simulink model "ipmsm_velocity_control_system_coupler"  (R2022a)
settings: Solver=daessc  StartTime=0.0  StopTime=SimStopTime  FixedStep=Ts  RelTol=1e-3  AbsTol=1e-3
values from neighbouring files (symbols this model uses):
  battery_pack_TimeStep = 0.01    [PMSM_system_data.sldd]
  Ts = 5.0E-6    [PMSM_system_data.sldd]
  V_init = 377.0    [PMSM_plant_parameters.sldd]
undefined symbols (not defined in the file or in its folder): DiscIntNeverNeededParam, iabc, rotation_speed, Tq, V_dc
libraries: fl_lib x20, nesl_utility x20, ee_lib x4, simulink x1, eePwmGeneratorTwoLevel x1, SignalEditorBlockLib x1
Description:
  | IPMSM Velocity Control
settings Model: DataDictionary=PMSM_system_data.sldd  Creator=The MathWorks, Inc.  LastModifiedBy=tshintai
settings SolverCC: AutoScaleAbsTol=off  AlgebraicLoopSolver=TrustRegion
settings DataIOCC: MaxDataPoints=210000  DSMLogging=off  SignalLoggingName=logsout_ee_ipmsm_velocity_control
settings OptimizationCC: LifeSpan=inf
settings DebuggingCC: UnderspecifiedInitializationDetection=Classic  MergeDetectMultiDrivingBlocksExec=none  ParameterPrecisionLossMsg=none  UnconnectedInputMsg=warning  UnconnectedOutputMsg=warning  UnconnectedLineMsg=warning  SFUnexpectedBacktrackingDiag=warning  SFNoUnconditionalDefaultTransitionDiag=warning  SFExecutionAtInitializationDiag=none  SFMachineParentedDataDiag=warning  ArithmeticOperatorsInVariantConditions=warning
settings SFSimCC: SimUseLocalCustomCode=off  CustomCodeUndefinedFunction=UseInterfaceOnly
settings RTWCC: RTWUseLocalCustomCode=off  DLArmComputeVersion=19.05
settings CodeAppCC: StateflowObjectComments=on
settings GRTTargetCC: TargetLangStandard=C89/C90 (ANSI)
settings ConfigComp: CovMetricSettings=dw  CovSaveCumulativeToWorkspaceVar=on  CovSaveSingleToWorkspaceVar=on  CovExternalEMLEnable=off
settings SimscapeCC: SimscapeNormalizeSystem=off  SimscapeLogType=all  SimscapeLogToSDI=on  SimscapeLogName=simlog_ee_ipmsm_velocity_control  SimscapeLogLimitData=off  SimscapeLogDataHistory=210000

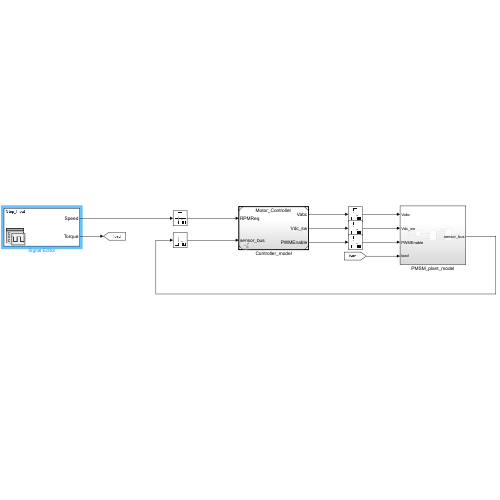
[thumbnail: Simulink's stored preview of the top-level diagram]
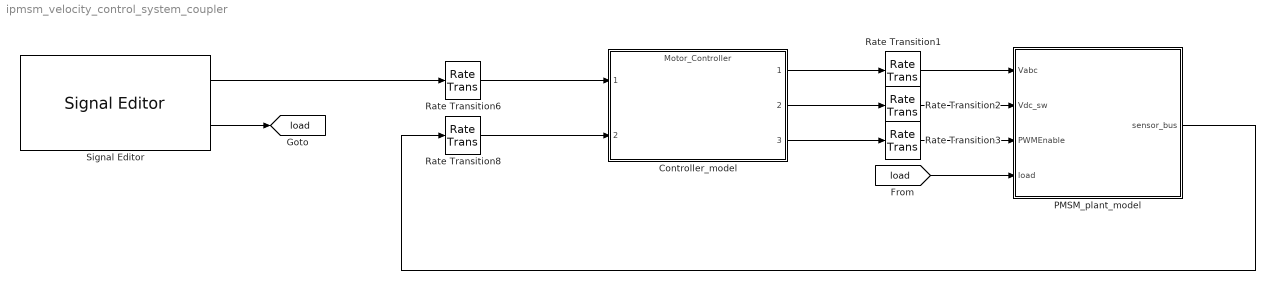
== system ipmsm_velocity_control_system_coupler ==
  Controller_model : ModelReference  ModelNameDialog=Motor_Controller.slx  SimulationMode=Normal  ModelReferenceVersion=4.3
  PMSM_plant_model : Subsystem
  Rate Transition1 : RateTransition
  Rate Transition2 : RateTransition
  Rate Transition3 : RateTransition
  Rate Transition6 : RateTransition  OutPortSampleTime=Tso
  Rate Transition8 : RateTransition  OutPortSampleTime=Tsi
  Signal Editor : SignalEditorBlockLib/Signal Editor  FileName=Motor_Controller_sig.mat  ActiveScenario=Step_Input  ActiveSignal=Speed  IsBus=off  OutputBusObjectStr=Bus: BusObject  SampleTime=0  ZeroCross=off  OutputAfterFinalValue=Holding final value  Unit=inherit  PreserveSignalName=on
  tag scope: load=global
  wires:
  Controller_model/1 -> Rate Transition1/1
  Signal Editor/2 -> [load]
  Signal Editor/1 -> Rate Transition6/1
  Rate Transition1/1 -> PMSM_plant_model/1(Vabc)
  Controller_model/2 -> Rate Transition2/1
  Rate Transition2/1 -> PMSM_plant_model/2(Vdc_sw)
  Rate Transition3/1 -> PMSM_plant_model/3(PWMEnable)
  Controller_model/3 -> Rate Transition3/1
  Rate Transition6/1 -> Controller_model/1
  [load] -> PMSM_plant_model/4(load)
  Rate Transition8/1 -> Controller_model/2
  PMSM_plant_model/1(sensor_bus) -> Rate Transition8/1

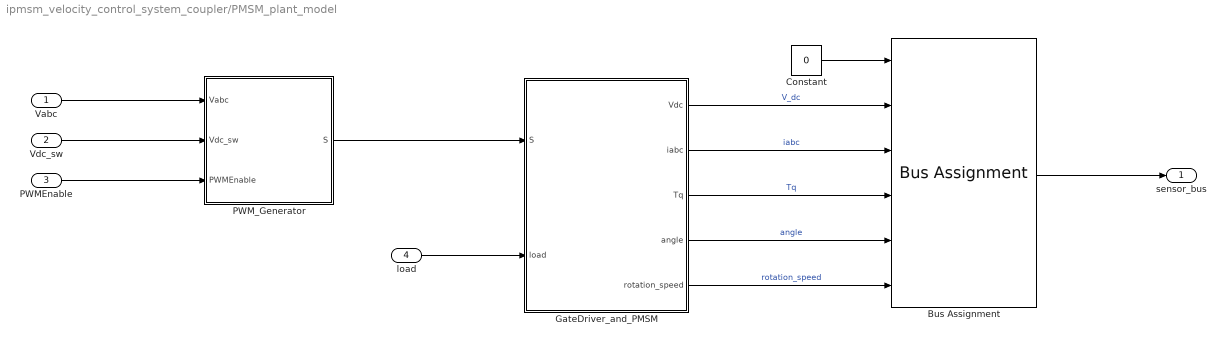
== system ipmsm_velocity_control_system_coupler/PMSM_plant_model ==
  Vabc : Inport
  Vdc_sw : Inport  Port=2
  PWMEnable : Inport  Port=3
  load : Inport  Port=4
  Bus Assignment : BusAssignment  AssignedSignals=V_dc,iabc,Tq,angle,rotation_speed
  Constant : Constant  Value=0  OutDataTypeStr=Bus: sensor_bus
  GateDriver_and_PMSM : Subsystem
  PWM_Generator : Subsystem
  sensor_bus : Outport
  wires:
  Vabc/1 -> PWM_Generator/1(Vabc)
  Vdc_sw/1 -> PWM_Generator/2(Vdc_sw)
  PWMEnable/1 -> PWM_Generator/3(PWMEnable)
  PWM_Generator/1(S) -> GateDriver_and_PMSM/1(S)
  load/1 -> GateDriver_and_PMSM/2(load)
  GateDriver_and_PMSM/1(Vdc) -> Bus Assignment/2  "V_dc"
  GateDriver_and_PMSM/2(iabc) -> Bus Assignment/3  "iabc"
  GateDriver_and_PMSM/3(Tq) -> Bus Assignment/4  "Tq"
  GateDriver_and_PMSM/4(angle) -> Bus Assignment/5  "angle"
  GateDriver_and_PMSM/5(rotation_speed) -> Bus Assignment/6  "rotation_speed"
  Constant/1 -> Bus Assignment/1
  Bus Assignment/1 -> sensor_bus/1

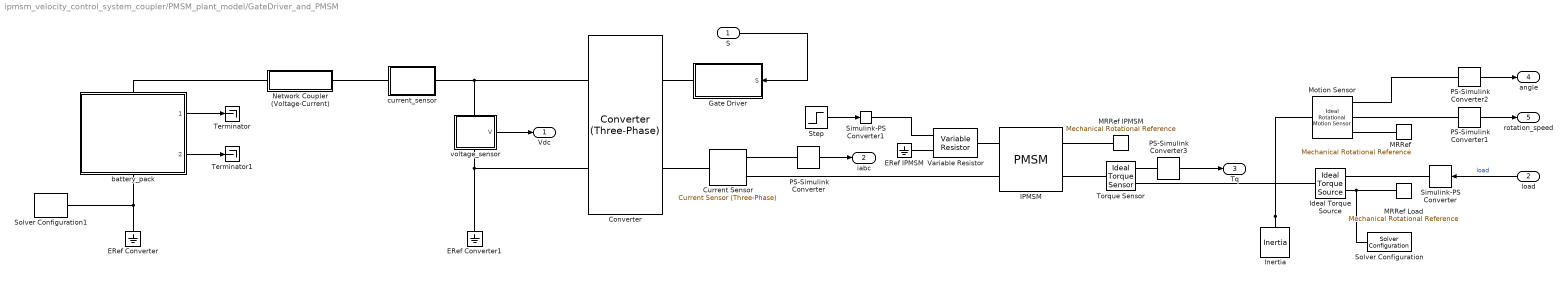
== system ipmsm_velocity_control_system_coupler/PMSM_plant_model/GateDriver_and_PMSM ==
  S : Inport
  load : Inport  Port=2
  Converter : ee_lib/Semiconductors & Converters/Converters/Converter (Three-Phase)  port_option=ee.enum.threePhasePort.composite  device_type=3  Vf=0.8 V  Ron=0.001 Ohm  Rds=0.001 Ohm  Goff=1e-5 1/Ohm  Vgt=1 V  Vgt_off=-1 V  Ih=1 A  Vth=0.5 V  diode_param=2  diode_Vf=0.8 V  diode_Ron=0.001 Ohm  diode_Goff=1e-5 1/Ohm  diode_C=50 nF  diode_iRM=-235 A  diode_iF=300 A  diode_idot=-50 A/us  diode_trr_param=1  diode_trr_factor=3  diode_trr=15 us  diode_Qrr=1.5e+3 s*uA  snubber_type=0  Cs=1e-7 F  Rs=0.1 Ohm
      settings: SourceProductBaseCode=PS
  Current Sensor : ee_lib/Sensors & Transducers/Current Sensor (Three-Phase)
  ERef Converter : fl_lib/Electrical/Electrical Elements/Electrical Reference
      settings: SourceProductBaseCode=PW,SS,VE
  ERef Converter1 : fl_lib/Electrical/Electrical Elements/Electrical Reference
      settings: SourceProductBaseCode=PW,SS,VE
  ERef IPMSM : fl_lib/Electrical/Electrical Elements/Electrical Reference
      settings: SourceProductBaseCode=PW,SS,VE
  Gate Driver : Subsystem
  IPMSM : ee_lib/Electromechanical/Permanent Magnet/PMSM  port_option=ee.enum.threePhasePort.composite  winding_type=ee.enum.statorconnection.wye  machine_param=ee.enum.pmsm.parameterization.constant  nPolePairs=p  pmflux_param=1  pm_flux_linkage=psim Wb  torque_constant=0.18 N*m/A  back_emf_constant=0.18 V/(rad/s)  stator_param=1  Ld=Ld H  Lq=Lq H  idVec=[-200, 0, 200] A  iqVec=[-200, 0, 200] A  LdMatrix=0.0002 * ones(3, 3) H  LqMatrix=0.0002 * ones(3, 3) H  PmMatrix=0.1 * ones(3, 3) Wb  ktMatrix=0.18 * ones(3, 3) N*m/A  keMatrix=0.18 * ones(3, 3) V/(rad/s)  L0=L0 H  Ls=0.0002 H  Lm=0.00002 H  Ms=0.00002 H  Rs=Rs Ohm  zero_sequence=ee.enum.park.zerosequence.include  axes_param=1  loss_param=ee.enum.ironloss.none  losses_oc=[0, 0, 0] W  losses_sc=[0, 0, 0] W  f_losses=60 Hz  Isc_losses=95 A  J=0 kg*m^2  lam=0 N*m/(rad/s)  i_d_specify=off  i_d_priority=None  i_d=0 A  i_d_nominal_specify=off  i_d_nominal_unit=A  i_d_nominal_value=1  i_q_specify=off  i_q_priority=None  i_q=0 A  i_q_nominal_specify=off  i_q_nominal_unit=A  i_q_nominal_value=1  torque_specify=off  torque_priority=None  torque=0 N*m  torque_nominal_specify=off  torque_nominal_unit=N*m  torque_nominal_value=1  angular_velocity_specify=on  angular_velocity_priority=None  angular_velocity=0 rpm  angular_velocity_nominal_specify=off  angular_velocity_nominal_unit=rpm  angular_velocity_nominal_value=1  angular_position_specify=on  angular_position_priority=High  angular_position=0 rad  angular_position_nominal_specify=off  angular_position_nominal_unit=deg  angular_position_nominal_value=1  alpha=3.93e-3 1/K  alpha_flux=-0.001 1/K  Tmeas=298.15 K  stator_thermal_mass=100 J/K  rotor_thermal_mass=200 J/K  Rm_percent_rotor=90  Rd_percent_rotor=30  temperatureA_specify=off  temperatureA_priority=High  temperatureA=25 degC  temperatureA_nominal_specify=off  temperatureA_nominal_unit=degC  temperatureA_nominal_value=1  temperatureB_specify=off  temperatureB_priority=High  temperatureB=25 degC  temperatureB_nominal_specify=off  temperatureB_nominal_unit=degC  temperatureB_nominal_value=1  temperatureC_specify=off  temperatureC_priority=High  temperatureC=25 degC  temperatureC_nominal_specify=off  temperatureC_nominal_unit=degC  temperatureC_nominal_value=1  temperatureR_specify=off  temperatureR_priority=High  temperatureR=25 degC  temperatureR_nominal_specify=off  temperatureR_nominal_unit=degC  temperatureR_nominal_value=1
      settings: AttributesFormatString=35 kW  InternalSimscapePortConfiguration="{\"Bottom\":[],\"Left\":[{\"id\":\"N\",\"label\":\"~\",\"type\":\"foundation.electrical.three_phase\"},{\"id\":\"n\",\"label\":\"n\",\"type\":\"foundation.electrical.electrical\"}],\"Right\":[{\"id\":\"R\",\"label\":\"R\",\"type\":\"foundation.mechanical.rotational.rotational\"},{\"id\":\"C\",\"label\":\"C\",\"type\":\"foundation.mechanical.rotational.rotational\"}],\"Top\":[]}"
  Ideal Torque Source : fl_lib/Mechanical/Mechanical Sources/Ideal Torque Source
      settings: SourceProductBaseCode=PW,SS,VE
  Inertia : fl_lib/Mechanical/Rotational Elements/Inertia  inertia=Jm kg*m^2  num_ports=foundation.enum.numPorts2.one  w_specify=on  w_priority=High  w=0 rpm  w_nominal_specify=off  w_nominal_unit=rad/s  w_nominal_value=1  t_specify=off  t_priority=High  t=0 N*m  t_nominal_specify=off  t_nominal_unit=N*m  t_nominal_value=1
      settings: SourceProductBaseCode=PW,SS,VE
  MRRef : fl_lib/Mechanical/Rotational Elements/Mechanical Rotational Reference
      settings: SourceProductBaseCode=PW,SS,VE
  MRRef IPMSM : fl_lib/Mechanical/Rotational Elements/Mechanical Rotational Reference
      settings: SourceProductBaseCode=PW,SS,VE
  MRRef Load : fl_lib/Mechanical/Rotational Elements/Mechanical Rotational Reference
      settings: SourceProductBaseCode=PW,SS,VE
  Motion Sensor : fl_lib/Mechanical/Mechanical Sensors/Ideal Rotational Motion Sensor  wrap_angle=simscape.enum.onoff.off  offset=0 deg
      settings: SourceProductBaseCode=PW,SS,VE
  Network Coupler (Voltage-Current) : Subsystem  mask(Network Coupler (Voltage-Current)){}
      mask init:
      | % Icon
      | key = 'Simscape.NetworkCouplers.ElectricalVoltageCurrent';
      | foundation.internal.couplers.updateIcon(gcb,'voltageCurrentSource.svg',key)
      settings: OpenFcn=open_system(gcbh,'force')
      mask Help: web([docroot '/physmod/simscape/ref/networkcouplervoltagecurrent.html'])
      mask Display:
      | color('red');
      | port_label('LConn', 1,'1')
      | port_label('RConn', 1,'2')
  PS-Simulink Converter : nesl_utility/PS-Simulink Converter  PhysicalDomain=network_engine_domain  SubClassName=ps_output  LeftPortType=input  RightPortType=output  PseudoPeriodic=off  Frequencies=[]  VectorFormat=1-D array  Unit=A  AffineConversion=off
      settings: SourceProductBaseCode=SS,PW,VE
  PS-Simulink Converter1 : nesl_utility/PS-Simulink Converter  PhysicalDomain=network_engine_domain  SubClassName=ps_output  LeftPortType=input  RightPortType=output  PseudoPeriodic=off  Frequencies=[]  VectorFormat=1-D array  Unit=rad/s  AffineConversion=off
      settings: SourceProductBaseCode=SS,PW,VE
  PS-Simulink Converter2 : nesl_utility/PS-Simulink Converter  PhysicalDomain=network_engine_domain  SubClassName=ps_output  LeftPortType=input  RightPortType=output  PseudoPeriodic=off  Frequencies=[]  VectorFormat=1-D array  Unit=rad  AffineConversion=off
      settings: SourceProductBaseCode=SS,PW,VE
  PS-Simulink Converter3 : nesl_utility/PS-Simulink Converter  PhysicalDomain=network_engine_domain  SubClassName=ps_output  LeftPortType=input  RightPortType=output  PseudoPeriodic=off  Frequencies=[]  VectorFormat=1-D array  Unit=N*m  AffineConversion=off
      settings: SourceProductBaseCode=SS,PW,VE
  Simulink-PS Converter : nesl_utility/Simulink-PS Converter  PhysicalDomain=network_engine_domain  SubClassName=ps_input  LeftPortType=input  RightPortType=output  PseudoPeriodic=off  Frequencies=[]  NoiseDistribution=none  NoiseParameters=[]  Unit=N*m  AffineConversion=off  FilteringAndDerivatives=zero  SimscapeFilterOrder=1  InputFilterTimeConstant=0.001  UdotUserProvided=1
      settings: SourceProductBaseCode=SS,PW,VE
  Simulink-PS Converter1 : nesl_utility/Simulink-PS Converter  PhysicalDomain=network_engine_domain  SubClassName=ps_input  LeftPortType=input  RightPortType=output  PseudoPeriodic=off  Frequencies=[]  NoiseDistribution=none  NoiseParameters=[]  Unit=1  AffineConversion=off  FilteringAndDerivatives=provide  SimscapeFilterOrder=1  InputFilterTimeConstant=0.001  UdotUserProvided=0
      settings: SourceProductBaseCode=SS,PW,VE
  Solver Configuration : nesl_utility/Solver Configuration  PhysicalDomain=network_engine_domain  SubClassName=solver  LeftPortType=input  RightPortType=generic  Tones=[]  Harmonics=[]  SimulateNoise=off  Profile=off  UseLocalSampling=off  EnableSwitchedLinearOptims=on  FrequencyDomain=off  UseCCode=off  RelTol=0.001  AbsTol=1e-06  MinStep=1e-09  ToWorkspace=off  RevertToSquareIcSolve=off  NumHomotopyIterations=100  PhasorMode=off  PhasorModeNumHarmonics=1  IndexReductionMethod=DerivativeReplacement  DoDC=off  ResidualTolerance=1e-9  UseLocalSolver=on  LocalSolverChoice=NE_BACKWARD_EULER_ADVANCER  LocalSolverSampleTime=Ts  DoFixedCost=on  MaxNonlinIter=5  MaxModeIter=2  ComputeImpulses=off  ImpulseIterations=2  LinearAlgebra=auto  LinearAlgebraNumThread=0  EquationFormulation=NE_TIME_EF  DelaysMemoryBudget=1024  AutomaticFiltering=on  FilteringTimeConstant=0.001  PartitionStorageMethod=AS_NEEDED  PartitionMemoryBudget=1024  PartitionMethod=FAST
      settings: SourceProductBaseCode=SS,PW,VE
  Solver Configuration1 : nesl_utility/Solver Configuration  PhysicalDomain=network_engine_domain  SubClassName=solver  LeftPortType=input  RightPortType=generic  Tones=[]  Harmonics=[]  SimulateNoise=off  Profile=off  UseLocalSampling=off  EnableSwitchedLinearOptims=on  FrequencyDomain=off  UseCCode=off  RelTol=0.001  AbsTol=0.001  MinStep=1e-09  ToWorkspace=off  RevertToSquareIcSolve=off  NumHomotopyIterations=100  PhasorMode=off  PhasorModeNumHarmonics=1  IndexReductionMethod=DerivativeReplacement  DoDC=off  ResidualTolerance=1e-09  UseLocalSolver=on  LocalSolverChoice=NE_BACKWARD_EULER_ADVANCER  LocalSolverSampleTime=battery_pack_TimeStep  DoFixedCost=on  MaxNonlinIter=3  MaxModeIter=2  ComputeImpulses=off  ImpulseIterations=2  LinearAlgebra=auto  LinearAlgebraNumThread=0  EquationFormulation=NE_TIME_EF  DelaysMemoryBudget=1024  AutomaticFiltering=on  FilteringTimeConstant=0.001  PartitionStorageMethod=AS_NEEDED  PartitionMemoryBudget=1024  PartitionMethod=ROBUST
      settings: SourceProductBaseCode=SS,PW,VE
  Step : Step  Time=0.3  Before=1e9  After=1e9  SampleTime=0
  Terminator : Terminator
  Terminator1 : Terminator
  Torque Sensor : fl_lib/Mechanical/Mechanical Sensors/Ideal Torque Sensor
      settings: SourceProductBaseCode=PW,SS,VE
  Variable Resistor : fl_lib/Electrical/Electrical Elements/Variable Resistor  Rmin=0 Ohm  i_specify=off  i_priority=None  i=0 A  i_nominal_specify=off  i_nominal_unit=A  i_nominal_value=1  v_specify=off  v_priority=None  v=0 V  v_nominal_specify=off  v_nominal_unit=V  v_nominal_value=1
      settings: SourceProductBaseCode=PW,SS,VE
  battery_pack : Subsystem  ReferencedSubsystem=battery_96_pack
      settings: PortSchema="{\"entries\":[{\"content\":{\"sides\":[{\"content\":{\"connectorIds\":[]},\"type\":\"ConnectorPlacement.EquallySpacedRectSide\",\"uuid\":\"485b780b-fec5-4a6e-9c4a-84b4d939a40e\"},{\"content\":{\"connectorIds\":[\"Out1\",\"Out2\"],\"side\":\"RIGHT\"},\"type\":\"ConnectorPlacement.EquallySpacedRectSide\",\"uuid\":\"e63a9d0c-46b2-44d5-a80a-3c6cfd714558\"},{\"content\":{\"connectorIds\":[\"LConn1\"],\"side\":\"TOP\"},\"type\":\"ConnectorPlacement.EquallySpacedRectSide\",\"uuid\":\"fa88f5e9-c256-49a0-983f-41440d45b27d\"},{\"content\":{\"connectorIds\":[\"RConn1\"],\"side\":\"BOTTOM\"},\"type\":\"ConnectorPlacement.EquallySpacedRectSide\",\"uuid\":\"af720e83-a3fc-4197-ae0f-d9d0aa453c8d\"}]},\"type\":\"ConnectorPlacement.EquallySpacedConnector\",\"uuid\":\"f46161be-ef35-45f2-922c-6cbb80c1717a\"}],\"packageUris\":[\"http://schema.mathworks.com/mf0/Connector/R2020b\"],\"version\":\"1.0\"}"
  current_sensor : Subsystem
  voltage_sensor : Subsystem
      settings: PortSchema="{\"entries\":[{\"content\":{\"sides\":[{\"content\":{\"connectorIds\":[]},\"type\":\"ConnectorPlacement.EquallySpacedRectSide\",\"uuid\":\"3cec5e81-2f0a-4a37-ad46-63204ea5d66a\"},{\"content\":{\"connectorIds\":[\"Out1\"],\"side\":\"RIGHT\"},\"type\":\"ConnectorPlacement.EquallySpacedRectSide\",\"uuid\":\"919246d8-ddc0-4701-8a0b-6f7af372975e\"},{\"content\":{\"connectorIds\":[\"LConn1\"],\"side\":\"TOP\"},\"type\":\"ConnectorPlacement.EquallySpacedRectSide\",\"uuid\":\"caca8a5a-fb83-489d-995f-a589d1d02c9f\"},{\"content\":{\"connectorIds\":[\"RConn1\"],\"side\":\"BOTTOM\"},\"type\":\"ConnectorPlacement.EquallySpacedRectSide\",\"uuid\":\"97d0da43-b632-476f-bdfd-058552dcf5f1\"}]},\"type\":\"ConnectorPlacement.EquallySpacedConnector\",\"uuid\":\"08c9aed4-62a1-4b8a-bec9-e16a3b517ce3\"}],\"packageUris\":[\"http://schema.mathworks.com/mf0/Connector/R2020b\"],\"version\":\"1.0\"}"
  Vdc : Outport
  iabc : Outport  Port=2
  Tq : Outport  Port=3
  angle : Outport  Port=4
  rotation_speed : Outport  Port=5
  wires:
  load/1 -> Simulink-PS Converter/1  "load"
  S/1 -> Gate Driver/1(S)
  PS-Simulink Converter/1 -> iabc/1
  PS-Simulink Converter2/1 -> angle/1
  PS-Simulink Converter1/1 -> rotation_speed/1
  PS-Simulink Converter3/1 -> Tq/1
  Step/1 -> Simulink-PS Converter1/1
  voltage_sensor/1(V) -> Vdc/1
  battery_pack/1 -> Terminator/1
  battery_pack/2 -> Terminator1/1
  connections:
  Variable Resistor/LConn2 -- ERef IPMSM/LConn1
  Ideal Torque Source/RConn1 -- Simulink-PS Converter/RConn1
  Variable Resistor/RConn1 -- IPMSM/LConn2
  Solver Configuration/RConn1 -- Ideal Torque Source/RConn2 -- MRRef Load/LConn1
  Gate Driver/RConn1 -- Converter/LConn1
  Torque Sensor/LConn1 -- IPMSM/RConn1
  Inertia/LConn1 -- Ideal Torque Source/LConn1 -- Torque Sensor/RConn1 -- Motion Sensor/LConn1
  Network Coupler (Voltage-Current)/LConn1 -- current_sensor/LConn1
  IPMSM/RConn2 -- MRRef IPMSM/LConn1
  Current Sensor/RConn1 -- PS-Simulink Converter/LConn1
  IPMSM/LConn1 -- Current Sensor/RConn2
  Converter/LConn2 -- Current Sensor/LConn1
  Motion Sensor/RConn2 -- PS-Simulink Converter1/LConn1
  Motion Sensor/RConn3 -- PS-Simulink Converter2/LConn1
  MRRef/LConn1 -- Motion Sensor/RConn1
  Torque Sensor/RConn2 -- PS-Simulink Converter3/LConn1
  Converter/RConn2 -- ERef Converter1/LConn1 -- voltage_sensor/RConn1
  Simulink-PS Converter1/RConn1 -- Variable Resistor/LConn1
  Converter/RConn1 -- voltage_sensor/LConn1 -- current_sensor/RConn1
  Network Coupler (Voltage-Current)/RConn1 -- battery_pack/LConn1
  Solver Configuration1/RConn1 -- ERef Converter/LConn1 -- battery_pack/RConn1

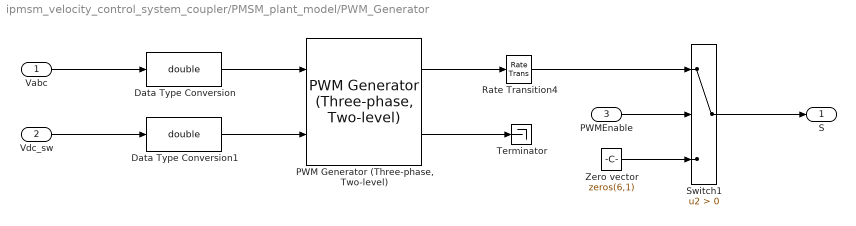
== system ipmsm_velocity_control_system_coupler/PMSM_plant_model/PWM_Generator ==
  Vabc : Inport
  Vdc_sw : Inport  Port=2
  PWMEnable : Inport  Port=3
  Data Type Conversion : DataTypeConversion  OutDataTypeStr=double  SaturateOnIntegerOverflow=off  RndMeth=Floor
  Data Type Conversion1 : DataTypeConversion  OutDataTypeStr=double  SaturateOnIntegerOverflow=off  RndMeth=Floor
  "PWM Generator (Three-phase, Two-level)" : eePwmGeneratorTwoLevel/PWM Generator (Three-phase, Two-level)  PWMMode=Continuous PWM (CPWM)  CPWMMode=SVM: space vector modulation  DPWMMode=60 DPWM: 60 degree discontinuous PWM  fsw=fsw  Ts=Ts
      settings: SourceProductBaseCode=PS
  Rate Transition4 : RateTransition
  Switch1 : Switch  Criteria=u2 > Threshold  SaturateOnIntegerOverflow=off  InputSameDT=off
  Terminator : Terminator
  Zero vector : Constant  Value=zeros(6,1)
  S : Outport
  wires:
  "PWM Generator (Three-phase, Two-level)"/2 -> Terminator/1
  Vabc/1 -> Data Type Conversion/1
  Zero vector/1 -> Switch1/3
  PWMEnable/1 -> Switch1/2
  Vdc_sw/1 -> Data Type Conversion1/1
  Rate Transition4/1 -> Switch1/1
  "PWM Generator (Three-phase, Two-level)"/1 -> Rate Transition4/1
  Switch1/1 -> S/1
  Data Type Conversion/1 -> "PWM Generator (Three-phase, Two-level)"/1
  Data Type Conversion1/1 -> "PWM Generator (Three-phase, Two-level)"/2

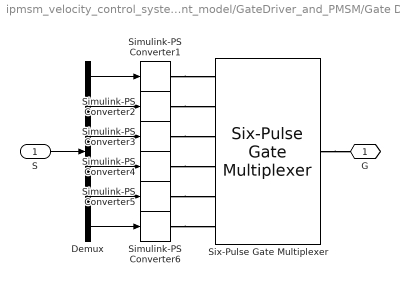
== system ipmsm_velocity_control_system_coupler/PMSM_plant_model/GateDriver_and_PMSM/Gate Driver ==
  S : Inport
  Demux : Demux  Outputs=6
  Simulink-PS Converter{1..6} (6 alike) : nesl_utility/Simulink-PS Converter  PhysicalDomain=network_engine_domain  SubClassName=ps_input  LeftPortType=input  RightPortType=output  PseudoPeriodic=off  Frequencies=[]  NoiseDistribution=none  NoiseParameters=[]  Unit=1  AffineConversion=off  FilteringAndDerivatives=zero  SimscapeFilterOrder=1  InputFilterTimeConstant=0.001  UdotUserProvided=1
      settings: SourceProductBaseCode=SS,PW,VE
  Six-Pulse Gate Multiplexer : ee_lib/Semiconductors & Converters/Converters/Six-Pulse Gate Multiplexer  port_option=ee.enum.controlport.ps
      settings: SourceProductBaseCode=PS
  G : PMIOPort  Side=Right
  wires:
  Demux/1 -> Simulink-PS Converter1/1
  S/1 -> Demux/1
  Demux/4 -> Simulink-PS Converter4/1
  Demux/2 -> Simulink-PS Converter2/1
  Demux/3 -> Simulink-PS Converter3/1
  Demux/5 -> Simulink-PS Converter5/1
  Demux/6 -> Simulink-PS Converter6/1
  connections:
  Six-Pulse Gate Multiplexer/RConn1 -- G/RConn1
  Simulink-PS Converter1/RConn1 -- Six-Pulse Gate Multiplexer/LConn1
  Simulink-PS Converter3/RConn1 -- Six-Pulse Gate Multiplexer/LConn3
  Simulink-PS Converter5/RConn1 -- Six-Pulse Gate Multiplexer/LConn5
  Simulink-PS Converter6/RConn1 -- Six-Pulse Gate Multiplexer/LConn6
  Simulink-PS Converter4/RConn1 -- Six-Pulse Gate Multiplexer/LConn4
  Simulink-PS Converter2/RConn1 -- Six-Pulse Gate Multiplexer/LConn2

== system ipmsm_velocity_control_system_coupler/PMSM_plant_model/GateDriver_and_PMSM/Network Coupler (Voltage-Current) ==
  note: Connect Port 1 to the network
      | with the smaller sample time, or
      | the network running variable step.
  note: Uncomment rate transition
      | blocks if one or both networks
      | are running fixed step.
  Port 1 Interface : Subsystem  mask(Network Coupler (Voltage-Current) Port 1 Interface){samplingType=Fixed step both ports with faster sampling at port 1, ts=1e-3, h1=Ts, h2=battery_pack_TimeStep, predictionDiscreteToContinuous=off, smoothingContinuousToDiscrete=off, predictionSlowToFast=off, smoothingFastToSlow=off, nSmooth=1, tsSmoothing=0.01, tsMax=0.5, tau=0.1, i0=0, v0=V_init}
      mask prompts: samplingType "physmod:simscape:couplers:SimscapeNetworkCouplersLib:SamplingType_MP"; ts "physmod:simscape:couplers:SimscapeNetworkCouplersLib:SeparatorTimeConstants_MP"; h1 "physmod:simscape:couplers:SimscapeNetworkCouplersLib:Port1NetworkDiscreteSampleTimes_MP"; h2 "physmod:simscape:couplers:SimscapeNetworkCouplersLib:Port2NetworkDiscreteSampleTimes_MP"; predictionDiscreteToContinuous "physmod:simscape:couplers:SimscapeNetworkCouplersLib:UsePredictionWhenConnectingFixedStepToVariableStep_MP"; smoothingContinuousToDiscrete "physmod:simscape:couplers:SimscapeNetworkCouplersLib:UseSmoothingWhenConnectingVariableStepToFixedStep_MP"; predictionSlowToFast "physmod:simscape:couplers:SimscapeNetworkCouplersLib:UsePredictionWhenConnectingSlowToFastSampleTimes_MP"; smoothingFastToSlow "physmod:simscape:couplers:SimscapeNetworkCouplersLib:UseSmoothingWhenConnectingFastToSlowSampleTimes_MP"; nSmooth "physmod:simscape:couplers:SimscapeNetworkCouplersLib:NumberOfSamplesOverWhichToSmooth_MP"; tsSmoothing "physmod:simscape:couplers:SimscapeNetworkCouplersLib:SmoothingTimeConstants_MP"; tsMax "physmod:simscape:couplers:SimscapeNetworkCouplersLib:CalculatedFastestTrackableTimeConstants_MP"; tau "physmod:simscape:couplers:SimscapeNetworkCouplersLib:CalculatedFilterTimeConstants_MP"; i0 "physmod:simscape:couplers:SimscapeNetworkCouplersLib:InitialCurrentA_MP"; v0 "physmod:simscape:couplers:SimscapeNetworkCouplersLib:InitialVoltageV_MP"
      mask help:
      | Port 1 interface for use when breaking two Simscape(TM) networks at an electrical connection. A first-order filter is used to break algebraic constraints between the two networks.
      |
      | Connect Port 1 to the network with the higher sample rate, or the network that is variable step if interfacing fixed step and variable step networks.
      mask init:
      | % Fixed step sample time value check
      | foundation.internal.couplers.checkSampleTimes(gcb,h1,h2);
      | 
      | % Derived parameters
      | [tau,tsMax] = foundation.internal.couplers.electrical.derivedParamsSources(gcb,ts,h1,h2);
      settings: PortSchema="{\"entries\":[{\"content\":{\"sides\":[{\"content\":{\"connectorIds\":[\"LConn1\"]},\"type\":\"ConnectorPlacement.EquallySpacedRectSide\",\"uuid\":\"a6d4a9fd-b5aa-40dc-ab7e-2b646b9b57bc\"},{\"content\":{\"connectorIds\":[\"Out1\",\"In1\"],\"side\":\"RIGHT\"},\"type\":\"ConnectorPlacement.EquallySpacedRectSide\",\"uuid\":\"31bb6273-5b9b-48d0-a1a2-6fbacb979b97\"},{\"content\":{\"connectorIds\":[],\"side\":\"TOP\"},\"type\":\"ConnectorPlacement.EquallySpacedRectSide\",\"uuid\":\"0f7afab2-4481-486c-9ad0-2b42c5b091a4\"}]},\"type\":\"ConnectorPlacement.EquallySpacedConnector\",\"uuid\":\"a98e47aa-cbfd-441a-b14c-c9ea515c056e\"}],\"packageUris\":[\"http://schema.mathworks.com/mf0/Connector/R2020b\"],\"version\":\"1.0\"}"
      mask Help: web([docroot '/physmod/simscape/ref/networkcouplervoltagecurrent.html'])
      mask TypeOptions samplingType: physmod:simscape:couplers:SimscapeNetworkCouplersLib:VariableStepAtPorts1And2_PV | physmod:simscape:couplers:SimscapeNetworkCouplersLib:VariableStepAtPort1AndFixedStepAtPort2_PV | physmod:simscape:couplers:SimscapeNetworkCouplersLib:FixedStepBothPortsWithCommonSampleTime_PV | physmod:simscape:couplers:SimscapeNetworkCouplersLib:FixedStepBothPortsWithFasterSamplingAtPort1_PV
      mask Callback samplingType: foundation.internal.couplers.electrical.parameterVisibilitiesSources(gcb)
      mask Callback predictionDiscreteToContinuous: foundation.internal.couplers.electrical.parameterVisibilitiesSources(gcb)
      mask Callback smoothingContinuousToDiscrete: foundation.internal.couplers.electrical.parameterVisibilitiesSources(gcb)
      mask Callback predictionSlowToFast: foundation.internal.couplers.electrical.parameterVisibilitiesSources(gcb)
      mask Callback smoothingFastToSlow: foundation.internal.couplers.electrical.parameterVisibilitiesSources(gcb)
      mask DialogControl Main Prompt: Main
      mask DialogControl samplingType Prompt: サンプリング タイプ
      mask DialogControl ts Prompt: 区切り時定数 (s)
      mask DialogControl h1 Prompt: 端子 1 のネットワークの離散サンプル時間 (s)
      mask DialogControl h2 Prompt: 端子 2 のネットワークの離散サンプル時間 (s)
      mask DialogControl predictionDiscreteToContinuous Prompt: 固定ステップを可変ステップに接続するときに予測を使用
      mask DialogControl smoothingContinuousToDiscrete Prompt: 可変ステップを固定ステップに接続するときに平滑化を使用
      mask DialogControl predictionSlowToFast Prompt: 低速のサンプル時間を高速のサンプル時間に接続するときに予測を使用
      mask DialogControl smoothingFastToSlow Prompt: 高速のサンプル時間を低速のサンプル時間に接続するときに平滑化を使用
      mask DialogControl nSmooth Prompt: 平滑化するサンプルの数
      mask DialogControl tsSmoothing Prompt: 平滑化時定数 (s)
      mask DialogControl Analysis Prompt: Analysis
      mask DialogControl tsMax Prompt: 計算された最速の追跡可能な時定数 (s)
      mask DialogControl tau Prompt: 計算されたフィルター時定数 (s)
      mask DialogControl updateRecommendations Prompt: Update
      mask DialogControl updateRecommendations Callback: foundation.internal.couplers.electrical.analysisSources(gcb);
      mask DialogControl InitialConditions Prompt: Initial Conditions
      mask DialogControl i0 Prompt: 初期電流 (A)
      mask DialogControl v0 Prompt: 初期電圧 (V)
  Port 2 Interface : Subsystem  mask(Network Coupler (Voltage-Current) Port 2 Interface){}
      mask help: physmod:simscape:couplers:SimscapeNetworkCouplersLib:NetworkCouplerVoltageCurrentPort2Interface_MD
      settings: PortSchema="{\"entries\":[{\"content\":{\"sides\":[{\"content\":{\"connectorIds\":[\"In1\",\"Out1\"]},\"type\":\"ConnectorPlacement.EquallySpacedRectSide\",\"uuid\":\"5a4c1550-e77d-42df-bf3e-b81963920de7\"},{\"content\":{\"connectorIds\":[\"RConn1\"],\"side\":\"RIGHT\"},\"type\":\"ConnectorPlacement.EquallySpacedRectSide\",\"uuid\":\"3fd730f7-5937-4563-a365-595aaae9027b\"},{\"content\":{\"connectorIds\":[],\"side\":\"TOP\"},\"type\":\"ConnectorPlacement.EquallySpacedRectSide\",\"uuid\":\"c16e04e4-26e8-4fd6-98d3-59adbef44c0d\"}]},\"type\":\"ConnectorPlacement.EquallySpacedConnector\",\"uuid\":\"5588d8d0-d459-45fe-a303-1ca6654e99d0\"}],\"packageUris\":[\"http://schema.mathworks.com/mf0/Connector/R2020b\"],\"version\":\"1.0\"}"
      mask Help: web([docroot '/physmod/simscape/ref/networkcouplervoltagecurrent.html'])
  Rate transition (fast-to-slow) : RateTransition  Commented=through  Integrity=off
  Rate transition (slow-to-fast) : RateTransition  Commented=through  Integrity=off
  1 : PMIOPort  Side=Left
  2 : PMIOPort  Port=2  Side=Right
  wires:
  Port 1 Interface/1(current) -> Rate transition (fast-to-slow)/1
  Rate transition (fast-to-slow)/1 -> Port 2 Interface/1(current)
  Port 2 Interface/1(voltage) -> Rate transition (slow-to-fast)/1
  Rate transition (slow-to-fast)/1 -> Port 1 Interface/1(voltage)
  connections:
  2/RConn1 -- Port 2 Interface/RConn1
  1/RConn1 -- Port 1 Interface/LConn1

== system ipmsm_velocity_control_system_coupler/PMSM_plant_model/GateDriver_and_PMSM/current_sensor ==
  Current Sensor1 : fl_lib/Electrical/Electrical Sensors/Current Sensor
      settings: SourceProductBaseCode=PW,SS,VE
  PS-Simulink Converter : nesl_utility/PS-Simulink Converter  PhysicalDomain=network_engine_domain  SubClassName=ps_output  LeftPortType=input  RightPortType=output  PseudoPeriodic=off  Frequencies=[]  VectorFormat=inherit  Unit=inherit  AffineConversion=off
      settings: SourceProductBaseCode=SS,PW,VE
  Terminator : Terminator
  + : PMIOPort  Side=Left
  - : PMIOPort  Port=2  Side=Right
  wires:
  PS-Simulink Converter/1 -> Terminator/1  "Idc"
  connections:
  PS-Simulink Converter/LConn1 -- Current Sensor1/RConn1
  Current Sensor1/LConn1 -- +/RConn1
  Current Sensor1/RConn2 -- -/RConn1

== system ipmsm_velocity_control_system_coupler/PMSM_plant_model/GateDriver_and_PMSM/voltage_sensor ==
  PS-Simulink Converter4 : nesl_utility/PS-Simulink Converter  PhysicalDomain=network_engine_domain  SubClassName=ps_output  LeftPortType=input  RightPortType=output  PseudoPeriodic=off  Frequencies=[]  VectorFormat=1-D array  Unit=V  AffineConversion=off
      settings: SourceProductBaseCode=SS,PW,VE
  Voltage Sensor : fl_lib/Electrical/Electrical Sensors/Voltage Sensor
      settings: SourceProductBaseCode=PW,SS,VE
  + : PMIOPort  Side=Left
  - : PMIOPort  Port=2  Side=Right
  V : Outport
  wires:
  PS-Simulink Converter4/1 -> V/1  "Vdc"
  connections:
  PS-Simulink Converter4/LConn1 -- Voltage Sensor/RConn1
  Voltage Sensor/LConn1 -- +/RConn1
  -/RConn1 -- Voltage Sensor/RConn2

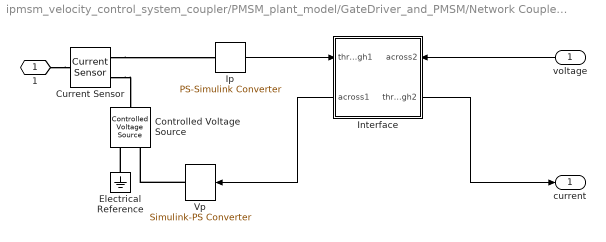
== system ipmsm_velocity_control_system_coupler/PMSM_plant_model/GateDriver_and_PMSM/Network Coupler (Voltage-Current)/Port 1 Interface ==
  voltage : Inport
  Controlled Voltage Source : fl_lib/Electrical/Electrical Sources/Controlled Voltage Source
      settings: SourceProductBaseCode=PW,SS,VE
  Current Sensor : fl_lib/Electrical/Electrical Sensors/Current Sensor
      settings: SourceProductBaseCode=PW,SS,VE
  Electrical Reference : fl_lib/Electrical/Electrical Elements/Electrical Reference
      settings: SourceProductBaseCode=PW,SS,VE
  Interface : Subsystem  Variant=on  VariantControlMode=label  VariantControl=Variant1  LabelModeActiveChoice=Discrete
      settings: PortSchema="{\"entries\":[{\"content\":{\"sides\":[{\"content\":{\"connectorIds\":[\"In1\",\"Out2\"]},\"type\":\"ConnectorPlacement.EquallySpacedRectSide\",\"uuid\":\"aa56821c-7799-44e3-b228-553c5b43a68d\"},{\"content\":{\"connectorIds\":[\"In2\",\"Out1\"],\"side\":\"RIGHT\"},\"type\":\"ConnectorPlacement.EquallySpacedRectSide\",\"uuid\":\"8658dee5-55e2-4f33-bdec-e6600ce27fc1\"},{\"content\":{\"connectorIds\":[],\"side\":\"TOP\"},\"type\":\"ConnectorPlacement.EquallySpacedRectSide\",\"uuid\":\"2effe9c6-8e61-4f0c-a39b-329d9ffc707d\"}]},\"type\":\"ConnectorPlacement.EquallySpacedConnector\",\"uuid\":\"c8fc8444-dfc7-49a5-9550-b957635f7d8f\"}],\"packageUris\":[\"http://schema.mathworks.com/mf0/Connector/R2020b\"],\"version\":\"1.0\"}"
  Ip : nesl_utility/PS-Simulink Converter  PhysicalDomain=network_engine_domain  SubClassName=ps_output  LeftPortType=input  RightPortType=output  PseudoPeriodic=off  Frequencies=[]  VectorFormat=1-D array  Unit=A  AffineConversion=off
      settings: SourceProductBaseCode=SS,PW,VE
  Vp : nesl_utility/Simulink-PS Converter  PhysicalDomain=network_engine_domain  SubClassName=ps_input  LeftPortType=input  RightPortType=output  PseudoPeriodic=off  Frequencies=[]  NoiseDistribution=none  NoiseParameters=[]  Unit=V  AffineConversion=off  FilteringAndDerivatives=zero  SimscapeFilterOrder=1  InputFilterTimeConstant=0.001  UdotUserProvided=1
      settings: SourceProductBaseCode=SS,PW,VE
  1 : PMIOPort  Side=Left
  current : Outport
  wires:
  Interface/1(through2) -> current/1
  Ip/1 -> Interface/1(through1)
  Interface/2(across1) -> Vp/1
  voltage/1 -> Interface/2(across2)
  connections:
  Electrical Reference/LConn1 -- Controlled Voltage Source/RConn2
  Current Sensor/RConn1 -- Ip/LConn1
  Current Sensor/RConn2 -- Controlled Voltage Source/LConn1
  1/RConn1 -- Current Sensor/LConn1
  Vp/RConn1 -- Controlled Voltage Source/RConn1

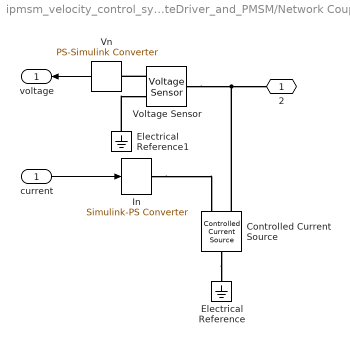
== system ipmsm_velocity_control_system_coupler/PMSM_plant_model/GateDriver_and_PMSM/Network Coupler (Voltage-Current)/Port 2 Interface ==
  current : Inport
  Controlled Current Source : fl_lib/Electrical/Electrical Sources/Controlled Current Source
      settings: SourceProductBaseCode=PW,SS,VE
  Electrical Reference : fl_lib/Electrical/Electrical Elements/Electrical Reference
      settings: SourceProductBaseCode=PW,SS,VE
  Electrical Reference1 : fl_lib/Electrical/Electrical Elements/Electrical Reference
      settings: SourceProductBaseCode=PW,SS,VE
  In : nesl_utility/Simulink-PS Converter  PhysicalDomain=network_engine_domain  SubClassName=ps_input  LeftPortType=input  RightPortType=output  PseudoPeriodic=off  Frequencies=[]  NoiseDistribution=none  NoiseParameters=[]  Unit=A  AffineConversion=off  FilteringAndDerivatives=zero  SimscapeFilterOrder=1  InputFilterTimeConstant=0.001  UdotUserProvided=1
      settings: SourceProductBaseCode=SS,PW,VE
  Vn : nesl_utility/PS-Simulink Converter  PhysicalDomain=network_engine_domain  SubClassName=ps_output  LeftPortType=input  RightPortType=output  PseudoPeriodic=off  Frequencies=[]  VectorFormat=1-D array  Unit=V  AffineConversion=off
      settings: SourceProductBaseCode=SS,PW,VE
  Voltage Sensor : fl_lib/Electrical/Electrical Sensors/Voltage Sensor
      settings: SourceProductBaseCode=PW,SS,VE
  2 : PMIOPort  Side=Right
  voltage : Outport
  wires:
  Vn/1 -> voltage/1
  current/1 -> In/1
  connections:
  Electrical Reference1/LConn1 -- Voltage Sensor/RConn2
  Voltage Sensor/LConn1 -- Controlled Current Source/RConn2 -- 2/RConn1
  Voltage Sensor/RConn1 -- Vn/LConn1
  Controlled Current Source/LConn1 -- Electrical Reference/LConn1
  In/RConn1 -- Controlled Current Source/RConn1

== system ipmsm_velocity_control_system_coupler/PMSM_plant_model/GateDriver_and_PMSM/Network Coupler (Voltage-Current)/Port 1 Interface/Interface ==
  through1 : Inport
  across2 : Inport  Port=2
  Continuous : Subsystem  VariantControl=Continuous
  Discrete : Subsystem  VariantControl=Discrete
  through2 : Outport
  across1 : Outport  Port=2

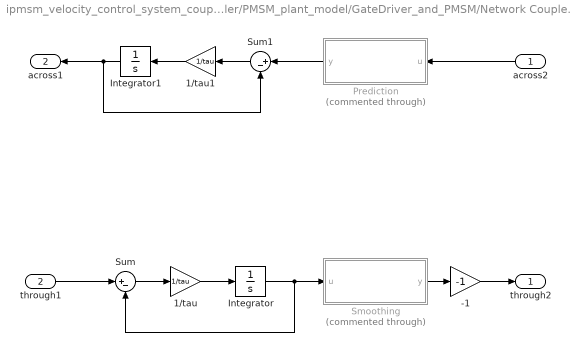
== system ipmsm_velocity_control_system_coupler/PMSM_plant_model/GateDriver_and_PMSM/Network Coupler (Voltage-Current)/Port 1 Interface/Interface/Continuous ==
  across2 : Inport
  through1 : Inport  Port=2
  -1 : Gain  Gain=-1  SaturateOnIntegerOverflow=on  OutDataTypeStr=Inherit: Same as input  ParamDataTypeStr=Inherit: Same as input
  1/tau : Gain  Gain=1/tau  SaturateOnIntegerOverflow=on  OutDataTypeStr=Inherit: Same as input  ParamDataTypeStr=Inherit: Same as input
  1/tau1 : Gain  Gain=1/tau  SaturateOnIntegerOverflow=on  OutDataTypeStr=Inherit: Same as input  ParamDataTypeStr=Inherit: Same as input
  Integrator : Integrator  InitialCondition=i0
  Integrator1 : Integrator  InitialCondition=v0
  Prediction : Subsystem  Commented=through  mask(Prediction (discrete->continuous)){h2=h2}
      mask prompts: h2 "physmod:simscape:couplers:SimscapeNetworkCouplersLib:PortUDiscreteSampleTimes_MP"
      mask help: physmod:simscape:couplers:SimscapeNetworkCouplersLib:Predictiondiscretecontinuous_MD
      mask DialogControl h2 Prompt: 端子 u の離散サンプル時間 (s)
  Smoothing : Subsystem  Commented=through  mask(Smoothing (continuous->discrete)){tsSmoothing=tsSmoothing, smoothing0=i0}
      mask prompts: tsSmoothing "physmod:simscape:couplers:SimscapeNetworkCouplersLib:SmoothingTimeConstants_MP"; smoothing0 "physmod:simscape:couplers:SimscapeNetworkCouplersLib:InitialOutput_MP"
      mask help: physmod:simscape:couplers:SimscapeNetworkCouplersLib:Smoothingcontinuousdiscrete_MD
      mask DialogControl tsSmoothing Prompt: 平滑化時定数 (s)
      mask DialogControl smoothing0 Prompt: 初期出力
  Sum : Sum  Inputs=|+-  InputSameDT=on  SaturateOnIntegerOverflow=on  OutDataTypeStr=Inherit: Same as first input
  Sum1 : Sum  Inputs=|+-  InputSameDT=on  SaturateOnIntegerOverflow=on  OutDataTypeStr=Inherit: Same as first input
  through2 : Outport
  across1 : Outport  Port=2
  wires:
  -1/1 -> through2/1
  Prediction/1(y) -> Sum1/1
  Sum1/1 -> 1/tau1/1
  1/tau1/1 -> Integrator1/1
  Integrator1/1 -> across1/1, Sum1/2
  through1/1 -> Sum/1
  Integrator/1 -> Sum/2, Smoothing/1(u)
  Sum/1 -> 1/tau/1
  1/tau/1 -> Integrator/1
  Smoothing/1(y) -> -1/1
  across2/1 -> Prediction/1(u)

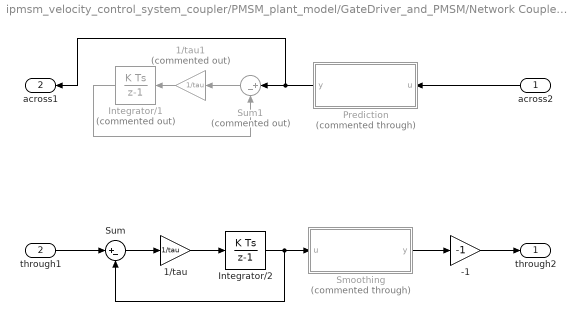
== system ipmsm_velocity_control_system_coupler/PMSM_plant_model/GateDriver_and_PMSM/Network Coupler (Voltage-Current)/Port 1 Interface/Interface/Discrete ==
  across2 : Inport
  through1 : Inport  Port=2
  -1 : Gain  Gain=-1  SaturateOnIntegerOverflow=on  OutDataTypeStr=Inherit: Same as input  ParamDataTypeStr=Inherit: Same as input
  1/tau : Gain  Gain=1/tau  SaturateOnIntegerOverflow=on  OutDataTypeStr=Inherit: Same as input  ParamDataTypeStr=Inherit: Same as input
  1/tau1 : Gain  Commented=on  Gain=1/tau  SaturateOnIntegerOverflow=on  OutDataTypeStr=Inherit: Same as input  ParamDataTypeStr=Inherit: Same as input
  Integrator/1 : DiscreteIntegrator  Commented=on  InitialCondition=v0  SampleTime=h1  ICPrevOutput=DiscIntNeverNeededParam  ICPrevScaledInput=DiscIntNeverNeededParam
  Integrator/2 : DiscreteIntegrator  InitialCondition=i0  SampleTime=h1  ICPrevOutput=DiscIntNeverNeededParam  ICPrevScaledInput=DiscIntNeverNeededParam
  Prediction : Subsystem  Commented=through  mask(Prediction (slow->fast)){h2=h2, h1=h1}
      mask prompts: h2 "physmod:simscape:couplers:SimscapeNetworkCouplersLib:PortUDiscreteSampleTimes_MP"; h1 "physmod:simscape:couplers:SimscapeNetworkCouplersLib:PortYDiscreteSampleTimes_MP"
      mask help: physmod:simscape:couplers:SimscapeNetworkCouplersLib:Predictionslowfast_MD
      mask DialogControl h2 Prompt: 端子 u の離散サンプル時間 (s)
      mask DialogControl h1 Prompt: 端子 y の離散サンプル時間 (s)
  Smoothing : Subsystem  Commented=through  mask(Smoothing (fast->slow)){nSmooth=nSmooth, h1=h1, smoothing0=i0}
      mask prompts: nSmooth "physmod:simscape:couplers:SimscapeNetworkCouplersLib:NumberOfSamplesOverWhichToSmooth_MP"; h1 "physmod:simscape:couplers:SimscapeNetworkCouplersLib:PortUDiscreteSampleTimes_MP"; smoothing0 "physmod:simscape:couplers:SimscapeNetworkCouplersLib:InitialOutput_MP"
      mask help: physmod:simscape:couplers:SimscapeNetworkCouplersLib:Smoothingfastslow_MD
      mask DialogControl nSmooth Prompt: 平滑化するサンプルの数
      mask DialogControl h1 Prompt: 端子 u の離散サンプル時間 (s)
      mask DialogControl smoothing0 Prompt: 初期出力
  Sum : Sum  Inputs=|+-  InputSameDT=on  SaturateOnIntegerOverflow=on  OutDataTypeStr=Inherit: Same as first input
  Sum1 : Sum  Commented=on  Inputs=|+-  InputSameDT=on  SaturateOnIntegerOverflow=on  OutDataTypeStr=Inherit: Same as first input
  through2 : Outport
  across1 : Outport  Port=2
  wires:
  -1/1 -> through2/1
  through1/1 -> Sum/1
  1/tau/1 -> Integrator/2/1
  1/tau1/1 -> Integrator/1/1
  Sum/1 -> 1/tau/1
  Integrator/2/1 -> Sum/2, Smoothing/1(u)
  Integrator/1/1 -> Sum1/2
  Sum1/1 -> 1/tau1/1
  Prediction/1(y) -> across1/1, Sum1/1
  Smoothing/1(y) -> -1/1
  across2/1 -> Prediction/1(u)

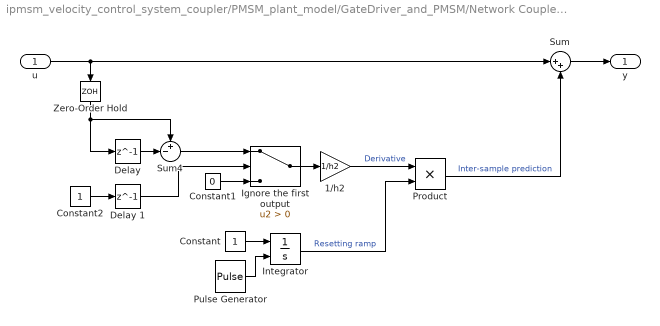
== system ipmsm_velocity_control_system_coupler/PMSM_plant_model/GateDriver_and_PMSM/Network Coupler (Voltage-Current)/Port 1 Interface/Interface/Continuous/Prediction ==
  u : Inport
  1/h2 : Gain  Gain=1/h2
  Constant : Constant  SampleTime=h2
  Constant1 : Constant  Value=0  SampleTime=h2
  Constant2 : Constant  SampleTime=h2
  "Delay " : Delay  DelayLength=1  SampleTime=h2
  Delay 1 : Delay  DelayLength=1  SampleTime=h2
  Ignore the first output : Switch  Criteria=u2 > Threshold  SaturateOnIntegerOverflow=off  InputSameDT=off
  Integrator : Integrator  ExternalReset=either  LimitOutput=on  UpperSaturationLimit=1  LowerSaturationLimit=0
  Product : Product
  Pulse Generator : DiscretePulseGenerator  SampleTime=h2
  Sum : Sum  Inputs=|++
  Sum4 : Sum  Inputs=+-|
  Zero-Order Hold : ZeroOrderHold  SampleTime=h2
  y : Outport
  wires:
  Constant2/1 -> Delay 1/1
  Delay 1/1 -> Ignore the first output/2
  Constant1/1 -> Ignore the first output/3
  Sum4/1 -> Ignore the first output/1
  Ignore the first output/1 -> 1/h2/1
  Pulse Generator/1 -> Integrator/2
  Constant/1 -> Integrator/1
  Integrator/1 -> Product/2  "Resetting ramp"
  Sum/1 -> y/1
  1/h2/1 -> Product/1  "Derivative"
  "Delay "/1 -> Sum4/2
  u/1 -> Zero-Order Hold/1, Sum/1
  Zero-Order Hold/1 -> "Delay "/1, Sum4/1
  Product/1 -> Sum/2  "Inter-sample prediction"

== system ipmsm_velocity_control_system_coupler/PMSM_plant_model/GateDriver_and_PMSM/Network Coupler (Voltage-Current)/Port 1 Interface/Interface/Continuous/Smoothing ==
  u : Inport
  Gain : Gain  Gain=1/tsSmoothing
  Integrator : Integrator  InitialCondition=smoothing0
  Sum : Sum  Inputs=|+-
  y : Outport
  wires:
  Sum/1 -> Gain/1
  Gain/1 -> Integrator/1
  Integrator/1 -> y/1, Sum/2
  u/1 -> Sum/1

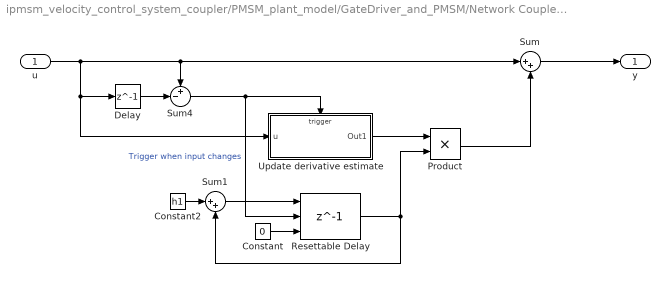
== system ipmsm_velocity_control_system_coupler/PMSM_plant_model/GateDriver_and_PMSM/Network Coupler (Voltage-Current)/Port 1 Interface/Interface/Discrete/Prediction ==
  u : Inport
  Constant : Constant  Value=0  SampleTime=h1
  Constant2 : Constant  Value=h1  SampleTime=h1
  "Delay " : Delay  DelayLength=1  SampleTime=h1
  Product : Product
  Resettable Delay : Delay  DelayLength=1  InitialConditionSource=Input port  ExternalReset=Rising  SampleTime=h1
      settings: InputPortMap=u0,r5,p4
  Sum : Sum  Inputs=|++
  Sum1 : Sum  Inputs=|++
  Sum4 : Sum  Inputs=+-|
  Update derivative estimate : Subsystem  TreatAsAtomicUnit=on
  y : Outport
  wires:
  Update derivative estimate/1(Out1) -> Product/1
  u/1 -> Sum/1, Sum4/1, Update derivative estimate/1(u), "Delay "/1
  "Delay "/1 -> Sum4/2
  Sum4/1 -> Update derivative estimate/Trigger, Resettable Delay/2  "Trigger when input changes"
  Sum1/1 -> Resettable Delay/1
  Resettable Delay/1 -> Product/2, Sum1/2
  Constant2/1 -> Sum1/1
  Constant/1 -> Resettable Delay/3
  Sum/1 -> y/1
  Product/1 -> Sum/2

== system ipmsm_velocity_control_system_coupler/PMSM_plant_model/GateDriver_and_PMSM/Network Coupler (Voltage-Current)/Port 1 Interface/Interface/Discrete/Smoothing ==
  u : Inport
  Gain : Gain  Gain=1/nSmooth
  Sum of Elements : Sum  Inputs=+
  Tapped Delay : simulink/Discrete/Tapped Delay  vinit=smoothing0  samptime=h1  NumDelays=nSmooth  DelayOrder=Oldest  includeCurrent=off
  y : Outport
  wires:
  u/1 -> Tapped Delay/1
  Tapped Delay/1 -> Sum of Elements/1
  Sum of Elements/1 -> Gain/1
  Gain/1 -> y/1

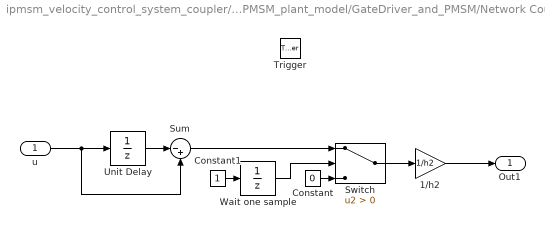
== system ipmsm_velocity_control_system_coupler/PMSM_plant_model/GateDriver_and_PMSM/Network Coupler (Voltage-Current)/Port 1 Interface/Interface/Discrete/Prediction/Update derivative estimate ==
  u : Inport
  Trigger : TriggerPort  VariantControl=(inherit)
  1/h2 : Gain  Gain=1/h2
  Constant : Constant  Value=0  SampleTime=-1
  Constant1 : Constant  SampleTime=-1
  Sum : Sum  Inputs=|-+
  Switch : Switch  Criteria=u2 > Threshold  SaturateOnIntegerOverflow=off  InputSameDT=off
  Unit Delay : UnitDelay  SampleTime=-1  HasFrameUpgradeWarning=on
  Wait one sample : UnitDelay  SampleTime=-1  HasFrameUpgradeWarning=on
  Out1 : Outport
  wires:
  Constant1/1 -> Wait one sample/1
  Wait one sample/1 -> Switch/2
  Constant/1 -> Switch/3
  Sum/1 -> Switch/1
  Switch/1 -> 1/h2/1
  1/h2/1 -> Out1/1
  u/1 -> Sum/2, Unit Delay/1
  Unit Delay/1 -> Sum/1
